simulink model "W2Q1"  (R2020b)
settings: Solver=VariableStepAuto  StartTime=0.0  StopTime=10.0  RelTol=1e-3
settings Model: Creator=HP  LastModifiedBy=HP

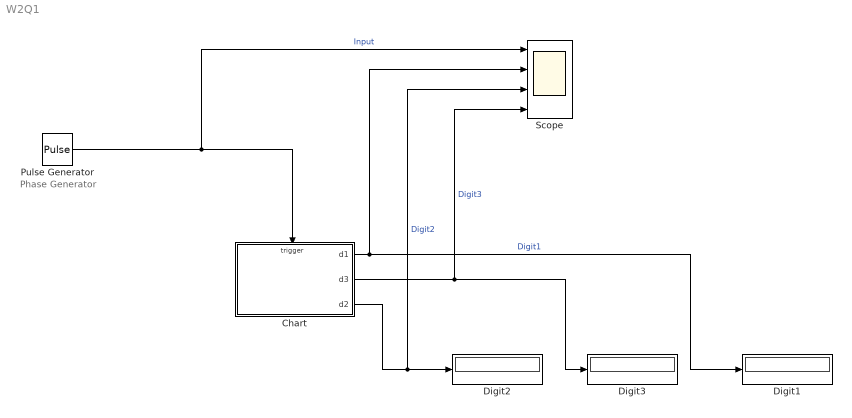
== system W2Q1 ==
  note: Phase Generator
  Chart : Stateflow chart  TreatAsAtomicUnit=on
  Digit1 : Display
  Digit2 : Display
  Digit3 : Display
  Pulse Generator : DiscretePulseGenerator  PulseType=Time based  Period=0.1  PulseWidth=5
  Scope : Scope  NumInputPorts=4
  wires:
  Chart/2(d3) -> Digit3/1, Scope/4  "Digit3"
  Pulse Generator/1 -> Scope/1, Chart/Trigger  "Input"
  Chart/3(d2) -> Scope/3, Digit2/1  "Digit2"
  Chart/1(d1) -> Scope/2, Digit1/1  "Digit1"

== stateflow chart W2Q1/Chart ==
  state digit1 [parallel]
    settings: executionOrder=1
    state One
      en:
      d1=1;
    state Two
      en:
      d1=2;
    state Three
      en:
      d1=3;
    state Zero
      en:
      d1=0;
    state Four
      en:
      d1=4;
    digit1.Three -> digit1.Four : in
    digit1.Two -> digit1.Three : in
    digit1.One -> digit1.Two : in
    digit1.Zero -> digit1.One : in
    (default) -> digit1.Zero
    digit1.Four -> digit1.Zero : in/{in2}
  state digit2 [parallel]
    settings: executionOrder=2
    state One
      en:
      d2=1;
    state Two
      en:
      d2=2;
    state Three
      en:
      d2=3;
    state Zero
      en:
      d2=0;
    state Four
      en:
      d2=4;
    digit2.Zero -> digit2.One : in2
    digit2.One -> digit2.Two : in2
    digit2.Two -> digit2.Three : in2
    digit2.Three -> digit2.Four : in2
    (default) -> digit2.Zero
    digit2.Four -> digit2.Zero : in2/{in3;}
  state digit3 [parallel]
    settings: executionOrder=3
    state One
      en:
      d3=1;
    state Two
      en:
      d3=2;
    state Three
      en:
      d3=3;
    state Zero
      en:
      d3=0;
    state Four
      en:
      d3=4;
    digit3.Three -> digit3.Four : in3
    digit3.Zero -> digit3.One : in3
    digit3.One -> digit3.Two : in3
    digit3.Two -> digit3.Three : in3
    (default) -> digit3.Zero
    digit3.Four -> digit3.Zero : in3
  data: d1 output; d3 output; d2 output
  events: in input EITHER_EDGE_EVENT; in2 local FUNCTION_CALL_EVENT; in3 local FUNCTION_CALL_EVENT
